simulink model "MonarcoHATdemo_task"  (Simulink 3.00)
libraries: mathlib x17, inoutlib x3, arclib x2

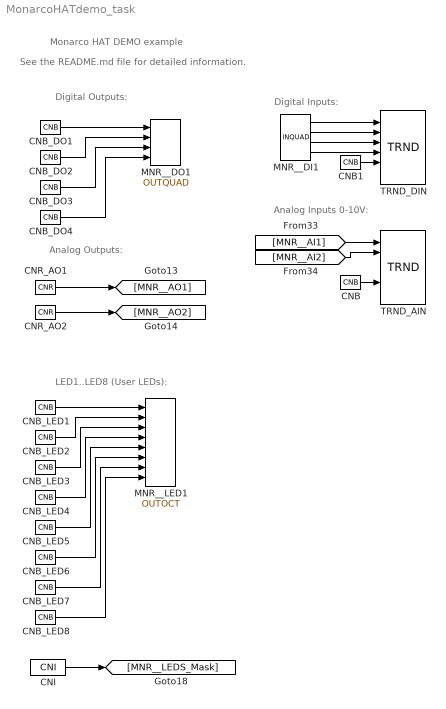
== system MonarcoHATdemo_task ==
  note: Analog Inputs 0-10V:
  note: Digital Inputs:
  note: Digital Outputs:
  note: Analog Outputs:
  note: LED1..LED8 (User LEDs):
  note: See the README.md file for detailed information.
  note: Monarco HAT DEMO example
  CNB : mathlib/CNB  YCN=on
  CNB1 : mathlib/CNB  YCN=on
  CNB_DO{1..4} (4 alike) : mathlib/CNB  YCN=off
  CNB_LED{1..8} (8 alike) : mathlib/CNB  YCN=off
  CNI : mathlib/CNI  icn=0x00
  CNR_AO1 : mathlib/CNR  ycn=0
  CNR_AO2 : mathlib/CNR  ycn=0
  MNR__DI1 : inoutlib/INQUAD
  MNR__DO1 : inoutlib/OUTQUAD
  MNR__LED1 : inoutlib/OUTOCT
  TRND_AIN : arclib/TRND  n=2  l=10000  btype=8: Double  ptype1=1: Store  ptype2=1: Store  ptype3=1: Store  ptype4=1: Store  pfac=1  afac=0  arc=0  id=1  Title=Trend Title  timesrc=1: CORETIMER
  TRND_DIN : arclib/TRND  n=4  l=10000  btype=8: Double  ptype1=1: Store  ptype2=1: Store  ptype3=1: Store  ptype4=1: Store  pfac=1  afac=0  arc=0  id=1  Title=Trend Title  timesrc=1: CORETIMER
  wires:
  CNB/1 -> TRND_AIN/5
  CNB1/1 -> TRND_DIN/5
  CNB_DO1/1 -> MNR__DO1/1
  CNB_DO2/1 -> MNR__DO1/2
  CNB_DO3/1 -> MNR__DO1/3
  CNB_DO4/1 -> MNR__DO1/4
  CNB_LED1/1 -> MNR__LED1/1
  CNB_LED2/1 -> MNR__LED1/2
  CNB_LED3/1 -> MNR__LED1/3
  CNB_LED4/1 -> MNR__LED1/4
  CNB_LED5/1 -> MNR__LED1/5
  CNB_LED6/1 -> MNR__LED1/6
  CNB_LED7/1 -> MNR__LED1/7
  CNB_LED8/1 -> MNR__LED1/8
  CNI/1 -> [MNR__LEDS_Mask]
  CNR_AO1/1 -> [MNR__AO1]
  CNR_AO2/1 -> [MNR__AO2]
  [MNR__AI1] -> TRND_AIN/1
  [MNR__AI2] -> TRND_AIN/2
  MNR__DI1/1 -> TRND_DIN/1
  MNR__DI1/2 -> TRND_DIN/2
  MNR__DI1/3 -> TRND_DIN/3
  MNR__DI1/4 -> TRND_DIN/4
